simulink model "teste2"  (R2020a)
settings: Solver=ode45  StartTime=0.0  StopTime=10  RelTol=1e-3
values from neighbouring files (symbols this model uses):
  d = 1.1    [constants.m]    (also in navigation.m = 0.64; path_plan.m = 1851851851.85; test_2w_sensor.m = 0.64)
  J = 1000    [constants.m]
  Kb = 0.06    [constants.m]
  ki = 66.99    [constants.m]
  kp = 38.15    [constants.m]
  Kt = 11.43    [constants.m]
  l = 0.64    [constants.m]
  L = 0.125    [constants.m]    (also in ekf_func_test.m = 2.2; kin_model.m = 2.2; model.m = 2.2; navigation.m = 2.2)
  m = 810    [constants.m]    (also in path_plan.m = numel(x_s))
  r = 0.256    [constants.m]    (also in navigation.m; test_2w_sensor.m)
  R = 0.688    [constants.m]    (also in ekf_func_test.m = [1 0 0 0; kin_controller.m = @(theta) [cos(theta),sin(theta),0;-sin(theta),cos(theta),0;0; test.m = 10*[1 0 0 0; test_2w.m = 10*[1 0 0)
libraries: simulink x3
settings Model: Creator=Tiago  LastModifiedBy=anapi
settings DebuggingCC: SFMachineParentedDataDiag=error

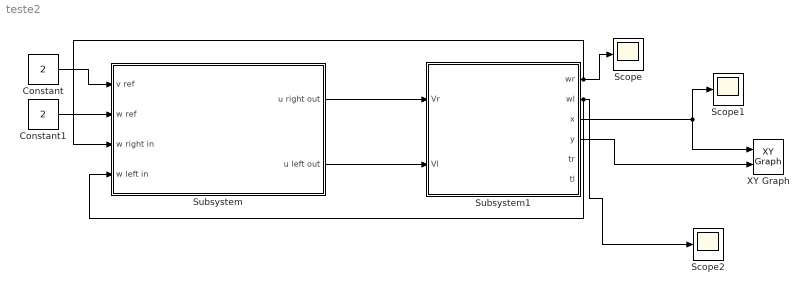
== system teste2 ==
  Constant : Constant  Value=2
  Constant1 : Constant  Value=2
  Scope : Scope
  Scope1 : Scope
  Scope2 : Scope
  Subsystem : Subsystem
  Subsystem1 : Subsystem
  XY Graph : simulink/Sinks/XY Graph  xmin=0  xmax=10  ymin=0  ymax=10  st=-1
  wires:
  Subsystem/2(u left out) -> Subsystem1/2(Vl)
  Subsystem/1(u right out) -> Subsystem1/1(Vr)
  Subsystem1/2(wl) -> Subsystem/4(w left in), Scope2/1
  Subsystem1/1(wr) -> Subsystem/3(w right in), Scope/1
  Subsystem1/3(x) -> XY Graph/1, Scope1/1
  Subsystem1/4(y) -> XY Graph/2
  Constant1/1 -> Subsystem/2(w ref)
  Constant/1 -> Subsystem/1(v ref)

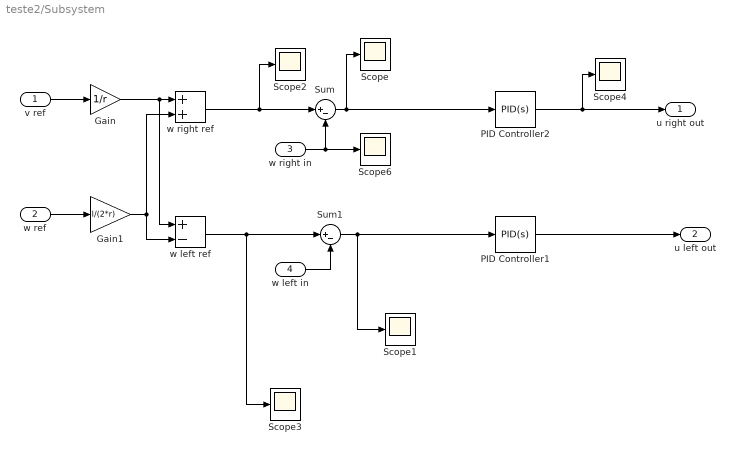
== system teste2/Subsystem ==
  v ref : Inport
  w ref : Inport  Port=2
  w right in : Inport  Port=3
  w left in : Inport  Port=4
  Gain : Gain  Gain=1/r
  Gain1 : Gain  Gain=l/(2*r)
  PID Controller1 : simulink/Continuous/PID Controller  Controller=PID  Form=Parallel  TimeDomain=Continuous-time  UseExternalTs=off  SampleTime=-1  IntegratorMethod=Forward Euler  FilterMethod=Forward Euler  ControllerParametersSource=internal  P=kp  I=ki  D=0  UseFilter=on  N=105296.504032148  TunerSelectOption=Transfer Function Based (PID Tuner App)  InitialConditionSource=internal  InitialConditionForIntegrator=0  InitialConditionForFilter=0  DifferentiatorICPrevScaledInput=0  ExternalReset=none  TrackingMode=off  Kt=1  LimitOutput=off  UpperSaturationLimit=inf  LowerSaturationLimit=-inf  LinearizeAsGain=on  AntiWindupMode=none  Kb=1  POutMin=[]  POutMax=[]  IOutMin=[]  IOutMax=[]  DOutMin=[]  DOutMax=[]  NOutMin=[]  NOutMax=[]  SumOutMin=[]  SumOutMax=[]  SaturationOutMin=[]  SaturationOutMax=[]  PParamMin=[]  PParamMax=[]  IParamMin=[]  IParamMax=[]  DParamMin=[]  DParamMax=[]  NParamMin=[]  NParamMax=[]  KbParamMin=[]  KbParamMax=[]  KtParamMin=[]  KtParamMax=[]  KbOutMin=[]  KbOutMax=[]  KtOutMin=[]  KtOutMax=[]  IntegratorOutMin=[]  IntegratorOutMax=[]  FilterOutMin=[]  FilterOutMax=[]  SumI1OutMin=[]  SumI1OutMax=[]  SumI2OutMin=[]  SumI2OutMax=[]  SumI3OutMin=[]  SumI3OutMax=[]  SumI4OutMin=[]  SumI4OutMax=[]  SumDOutMin=[]  SumDOutMax=[]  DifferentiatorOutMin=[]  DifferentiatorOutMax=[]  FilterDiffOutCoefMin=[]  FilterDiffOutCoefMax=[]  ReciprocalOutMin=[]  ReciprocalOutMax=[]  SumDenOutMin=[]  SumDenOutMax=[]  SumNumOutMin=[]  SumNumOutMax=[]  DivideOutMin=[]  DivideOutMax=[]  UdiffTsProdOutMin=[]  UdiffTsProdOutMax=[]  NTsProdOutMin=[]  NTsProdOutMax=[]  UintegralTsProdOutMin=[]  UintegralTsProdOutMax=[]  UngainTsProdOutMin=[]  UngainTsProdOutMax=[]  IntegratorContinuousStateAttributes=''  IntegratorStateMustResolveToSignalObject=off  IntegratorRTWStateStorageClass=Auto  FilterContinuousStateAttributes=''  FilterStateMustResolveToSignalObject=off  FilterRTWStateStorageClass=Auto  ParallelPVariant=InternalParameters  IdealPVariant=Disabled  IVariant=InternalParameters  DVariant=InternalParameters  IntegratorVariant=Continuous  SatVariant=Disabled  AWVariant=Passthrough  PCopyVariant=Disabled  TRVariant=Disabled  FdbkBlocksVariant=Forward  IdealPFdbkVariant=Disabled  SatFdbkVariant=Disabled  DerivativeFilterVariant=ContFilter  NVariant=InternalParameters  NCopyVariant=Disabled  FilterICVariant=InternalICsFilter  IntegratorICVariant=InternalICs  ExternalResetVariant=Disabled  TRSumVariant=Passthrough  SumFdbkVariant=Disabled  SumVariant=Sum_PID  TsampFilterVariant=InternalTs  TsampNgainVariant=Passthrough  TsampIntegralVariant=Passthrough
  PID Controller2 : simulink/Continuous/PID Controller  Controller=PID  Form=Parallel  TimeDomain=Continuous-time  UseExternalTs=off  SampleTime=-1  IntegratorMethod=Forward Euler  FilterMethod=Forward Euler  ControllerParametersSource=internal  P=ki  I=kp  D=0  UseFilter=on  N=105296.504032148  TunerSelectOption=Transfer Function Based (PID Tuner App)  InitialConditionSource=internal  InitialConditionForIntegrator=0  InitialConditionForFilter=0  DifferentiatorICPrevScaledInput=0  ExternalReset=none  TrackingMode=off  Kt=1  LimitOutput=off  UpperSaturationLimit=inf  LowerSaturationLimit=-inf  LinearizeAsGain=on  AntiWindupMode=none  Kb=1  POutMin=[]  POutMax=[]  IOutMin=[]  IOutMax=[]  DOutMin=[]  DOutMax=[]  NOutMin=[]  NOutMax=[]  SumOutMin=[]  SumOutMax=[]  SaturationOutMin=[]  SaturationOutMax=[]  PParamMin=[]  PParamMax=[]  IParamMin=[]  IParamMax=[]  DParamMin=[]  DParamMax=[]  NParamMin=[]  NParamMax=[]  KbParamMin=[]  KbParamMax=[]  KtParamMin=[]  KtParamMax=[]  KbOutMin=[]  KbOutMax=[]  KtOutMin=[]  KtOutMax=[]  IntegratorOutMin=[]  IntegratorOutMax=[]  FilterOutMin=[]  FilterOutMax=[]  SumI1OutMin=[]  SumI1OutMax=[]  SumI2OutMin=[]  SumI2OutMax=[]  SumI3OutMin=[]  SumI3OutMax=[]  SumI4OutMin=[]  SumI4OutMax=[]  SumDOutMin=[]  SumDOutMax=[]  DifferentiatorOutMin=[]  DifferentiatorOutMax=[]  FilterDiffOutCoefMin=[]  FilterDiffOutCoefMax=[]  ReciprocalOutMin=[]  ReciprocalOutMax=[]  SumDenOutMin=[]  SumDenOutMax=[]  SumNumOutMin=[]  SumNumOutMax=[]  DivideOutMin=[]  DivideOutMax=[]  UdiffTsProdOutMin=[]  UdiffTsProdOutMax=[]  NTsProdOutMin=[]  NTsProdOutMax=[]  UintegralTsProdOutMin=[]  UintegralTsProdOutMax=[]  UngainTsProdOutMin=[]  UngainTsProdOutMax=[]  IntegratorContinuousStateAttributes=''  IntegratorStateMustResolveToSignalObject=off  IntegratorRTWStateStorageClass=Auto  FilterContinuousStateAttributes=''  FilterStateMustResolveToSignalObject=off  FilterRTWStateStorageClass=Auto  ParallelPVariant=InternalParameters  IdealPVariant=Disabled  IVariant=InternalParameters  DVariant=InternalParameters  IntegratorVariant=Continuous  SatVariant=Disabled  AWVariant=Passthrough  PCopyVariant=Disabled  TRVariant=Disabled  FdbkBlocksVariant=Forward  IdealPFdbkVariant=Disabled  SatFdbkVariant=Disabled  DerivativeFilterVariant=ContFilter  NVariant=InternalParameters  NCopyVariant=Disabled  FilterICVariant=InternalICsFilter  IntegratorICVariant=InternalICs  ExternalResetVariant=Disabled  TRSumVariant=Passthrough  SumFdbkVariant=Disabled  SumVariant=Sum_PID  TsampFilterVariant=InternalTs  TsampNgainVariant=Passthrough  TsampIntegralVariant=Passthrough
  Scope{,1..4,6} (6 alike) : Scope
  Sum : Sum  Inputs=|+-
  Sum1 : Sum  Inputs=|+-
  w left ref : Sum  Inputs=+-
  w right ref : Sum
  u right out : Outport
  u left out : Outport  Port=2
  wires:
  v ref/1 -> Gain/1
  Gain/1 -> w right ref/1, w left ref/1
  Gain1/1 -> w right ref/2, w left ref/2
  w right ref/1 -> Scope2/1, Sum/1
  w left ref/1 -> Scope3/1, Sum1/1
  w right in/1 -> Scope6/1, Sum/2
  w left in/1 -> Sum1/2
  Sum/1 -> PID Controller2/1, Scope/1
  Sum1/1 -> PID Controller1/1, Scope1/1
  w ref/1 -> Gain1/1
  PID Controller2/1 -> Scope4/1, u right out/1
  PID Controller1/1 -> u left out/1

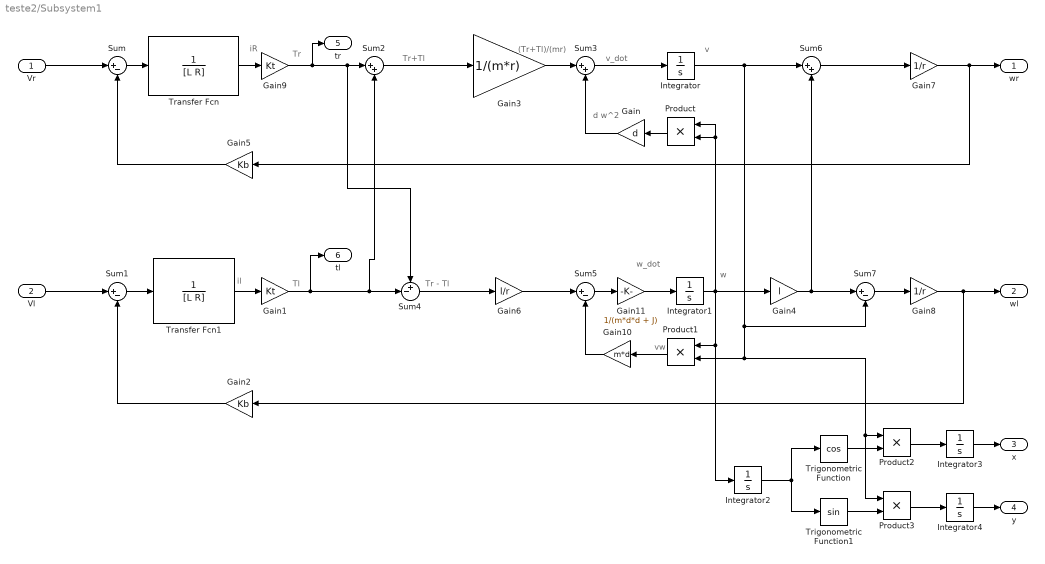
== system teste2/Subsystem1 ==
  note: Tr - Tl
  note: vw
  note: d w^2
  note: v
  note: il
  note: Tr+Tl
  note: w_dot
  note: Tr
  note: (Tr+Tl)/(mr)
  note: v_dot
  note: w
  note: iR
  note: Tl
  Vr : Inport
  Vl : Inport  Port=2
  Gain : Gain  Gain=d
  Gain1 : Gain  Gain=Kt
  Gain10 : Gain  Gain=m*d
  Gain11 : Gain  Gain=1/(m*d*d + J)
  Gain2 : Gain  Gain=Kb
  Gain3 : Gain  Gain=1/(m*r)
  Gain4 : Gain  Gain=l
  Gain5 : Gain  Gain=Kb
  Gain6 : Gain  Gain=l/r
  Gain7 : Gain  Gain=1/r
  Gain8 : Gain  Gain=1/r
  Gain9 : Gain  Gain=Kt
  Integrator{,1..4} (5 alike) : Integrator
  Product{,1..3} (4 alike) : Product
  Sum{,1,5,7} (4 alike) : Sum  Inputs=|+-
  Sum2 : Sum  Inputs=|++
  Sum3 : Sum  Inputs=|++
  Sum4 : Sum  Inputs=+-|
  Sum6 : Sum  Inputs=|++
  Transfer Fcn : TransferFcn  Denominator=[L R]
  Transfer Fcn1 : TransferFcn  Denominator=[L R]
  Trigonometric Function : Trigonometry  Operator=cos
  Trigonometric Function1 : Trigonometry
  wr : Outport
  wl : Outport  Port=2
  x : Outport  Port=3
  y : Outport  Port=4
  tr : Outport  Port=5
  tl : Outport  Port=6
  wires:
  Gain/1 -> Sum3/2
  Gain8/1 -> Gain2/1, wl/1
  Product1/1 -> Gain10/1
  Sum1/1 -> Transfer Fcn1/1
  Gain7/1 -> Gain5/1, wr/1
  Product/1 -> Gain/1
  Sum5/1 -> Gain11/1
  Gain10/1 -> Sum5/2
  Gain3/1 -> Sum3/1
  Gain11/1 -> Integrator1/1
  Sum7/1 -> Gain8/1
  Sum2/1 -> Gain3/1
  Sum6/1 -> Gain7/1
  Integrator/1 -> Sum6/1, Product3/1, Product2/1, Product1/2, Sum7/2
  Vl/1 -> Sum1/1
  Sum3/1 -> Integrator/1
  Gain6/1 -> Sum5/1
  Gain4/1 -> Sum7/1, Sum6/2
  Transfer Fcn1/1 -> Gain1/1
  Sum/1 -> Transfer Fcn/1
  Vr/1 -> Sum/1
  Integrator1/1 -> Integrator2/1, Product1/1, Gain4/1, Product/1, Product/2
  Transfer Fcn/1 -> Gain9/1
  Integrator2/1 -> Trigonometric Function1/1, Trigonometric Function/1
  Trigonometric Function/1 -> Product2/2
  Trigonometric Function1/1 -> Product3/2
  Product3/1 -> Integrator4/1
  Product2/1 -> Integrator3/1
  Integrator3/1 -> x/1
  Integrator4/1 -> y/1
  Sum4/1 -> Gain6/1
  Gain1/1 -> tl/1, Sum2/2, Sum4/2
  Gain9/1 -> tr/1, Sum4/1, Sum2/1
  Gain5/1 -> Sum/2
  Gain2/1 -> Sum1/2
